simulink model "Model_Excel"  (R2020a)
settings: Solver=VariableStepAuto  StartTime=0.0  StopTime=inf  RelTol=1e-3
model workspace (MAT data in the model file):
  WinSize = 16
  fc_bandpass = [0.05 0.25]
undefined symbols (not defined in the file or in its folder): A1, A104210, D1, P104210, W1, W104210
libraries: gtecHighspeedLib x1, dspsigops x1, dspfdesign x1, dspstat3 x1
(part 1 of 2)
settings Model: Creator=LAB-OREN3  LastModifiedBy=LAB-OREN3

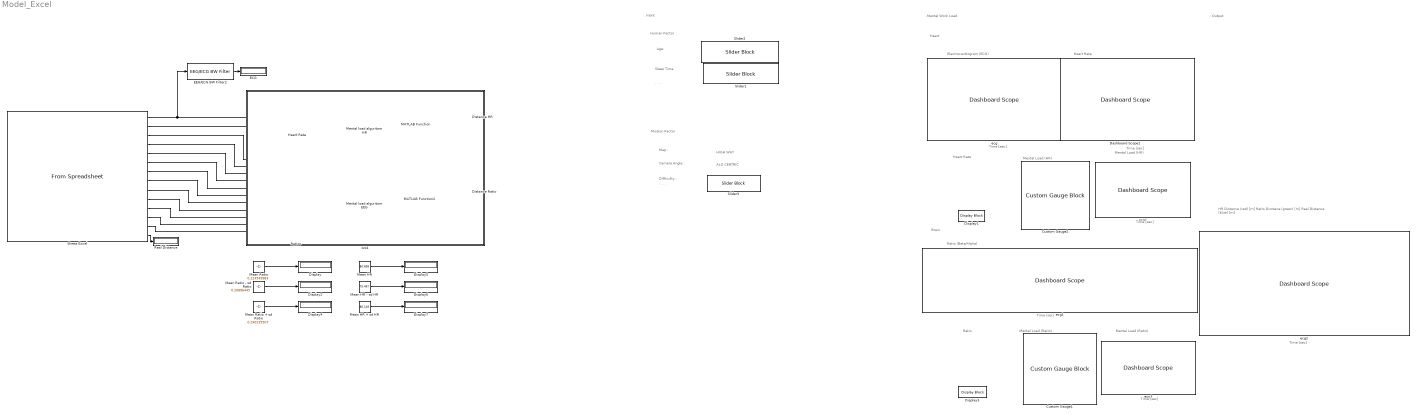
== system Model_Excel ==
  note: Time [sec]
  note: Heart Rate
  note: Mission Factor
  note: Ratio (Beta/Alpha)
  note: Electrocardiogram (ECG)
  note: Time (sec)
  note: Mental Load (Ratio)
  note: HIGH WAY
  note: Ratio
  note: ALO CENTRIC
  note: . Input
  note: Heart
  note: Time [sec]
  note: Sleep Time
  note: Human Factor
  note: Age:
  note: . Output
  note: Camera Angle: :
  note: . Mental Work Load
  note: Heart Rate
  note: Time [sec]
  note: Time [sec]
  note: Difficulty :
  note: .
      | .
      | .
      | .
  note: Brain
  note: Map :
  note: Time [sec]
  note: HR Distance (red) [m]
      | Ratio Disntace (green) [m]
      | Real Distance (blue) [m]
  note: .
      | .
      | .
      | .
  note: Mental Load (HR)
  note: Mental Load (Ratio)
  note: Mental Load (HR)
  Custom Gauge1 : CustomGaugeBlock  LabelPosition=Hide  NeedleImage=data:image/svg+xml;base64,PD94bWwgdmVyc2lvbj0iMS4wIiBlbmNvZGluZz0idXRmLTgiPz4KPCEtLSBHZW5lcmF0b3I6IEFkb2JlIElsbHVzdHJhdG9yIDE5LjIuMSwgU1ZHIEV4cG9ydCBQbHVnLUluIC4gU1ZHIFZlcnNpb246IDYuMDAgQnVpbGQgMCkgIC0tPgo8c3ZnIHZlcnNpb249IjEuMSIgeG1sbnM9Imh0dHA6Ly93d3cudzMub3JnLzIwMDAvc3ZnIiB4bWxuczp4bGluaz0iaHR0cDovL3d3dy53My5vcmcvMTk5OS94bGluayIgeD0iMHB4IiB5PSIwcHgiCgkgdmlld0JveD0iMCAwIDIwMCA1MCIgc3R5bGU9ImVuYWJsZS1iYWNrZ3JvdW5kOm5ldyAw ...(+9940 chars)  NeedleXPos=0.35442444142305646  NeedleYPos=0.4771166528829023  NeedleHeight=0.14101922133597494  NeedleWidth=0.2323187540223344  NeedleInitialRotation=-59.94322499147643  BackgroundImage=data:image/svg+xml;base64,PD94bWwgdmVyc2lvbj0iMS4wIiBlbmNvZGluZz0iVVRGLTgiIHN0YW5kYWxvbmU9Im5vIj8+CjwhLS0gR2VuZXJhdG9yOiBBZG9iZSBJbGx1c3RyYXRvciAxOS4yLjEsIFNWRyBFeHBvcnQgUGx1Zy1JbiAuIFNWRyBWZXJzaW9uOiA2LjAwIEJ1aWxkIDApICAtLT4KCjxzdmcKICAgeG1sbnM6ZGM9Imh0dHA6Ly9wdXJsLm9yZy9kYy9lbGVtZW50cy8xLjEvIgogICB4bWxuczpjYz0iaHR0cDovL2NyZWF0aXZlY29tbW9ucy5vcmcvbnMjIgogICB4bWxuczpyZGY9Imh0dHA6Ly93d3cudzMub3JnLzE5OTkvMDIvMjItcmRmLXN5bnRh ...(+9660 chars)  GaugeMax=1  GaugeArcDefined=true  GaugeArcRadius=0.16512766301399787  GaugeArcStrokeWidth=0.04828970295350007  GaugeArcRotation=240.5385250290321  GaugeArcRatio=0.8333333333333  GaugeArcTransparency=0  ValueArcTransparency=0  ValueArcColor=#1759b0  GaugeTickTransparency=0.55  GaugeTickColor=#faf5c8  ScaleColorsJSON="[{\"Min\":0,\"Max\":0.4,\"Color\":[0.39215686274509803,0.83137254901960778,0.074509803921568626]},{\"Min\":0.4,\"Max\":0.7,\"Color\":[0.92941176470588238,0.69411764705882351,0.12549019607843137]},{\"Min\":0.7,\"Max\":1,\"Color\":[0.996078431372549,0.2,0.0392156862745098]}]"  fixedAspectRatio=on  IsLinearGauge=false  GaugeTrackLeft=0.35  GaugeTrackTop=0.35  GaugeTrackHeight=0.1  GaugeTrackWidth=0.3  GaugeTrackRotation=0
  Custom Gauge2 : CustomGaugeBlock  LabelPosition=Hide  NeedleImage=data:image/svg+xml;base64,PD94bWwgdmVyc2lvbj0iMS4wIiBlbmNvZGluZz0idXRmLTgiPz4KPCEtLSBHZW5lcmF0b3I6IEFkb2JlIElsbHVzdHJhdG9yIDE5LjIuMSwgU1ZHIEV4cG9ydCBQbHVnLUluIC4gU1ZHIFZlcnNpb246IDYuMDAgQnVpbGQgMCkgIC0tPgo8c3ZnIHZlcnNpb249IjEuMSIgeG1sbnM9Imh0dHA6Ly93d3cudzMub3JnLzIwMDAvc3ZnIiB4bWxuczp4bGluaz0iaHR0cDovL3d3dy53My5vcmcvMTk5OS94bGluayIgeD0iMHB4IiB5PSIwcHgiCgkgdmlld0JveD0iMCAwIDIwMCA1MCIgc3R5bGU9ImVuYWJsZS1iYWNrZ3JvdW5kOm5ldyAw ...(+9940 chars)  NeedleXPos=0.3499172390096674  NeedleYPos=0.47640815567113937  NeedleHeight=0.14538535381695605  NeedleWidth=0.2395116348811877  NeedleInitialRotation=-59.94322499147643  BackgroundImage=data:image/svg+xml;base64,PD94bWwgdmVyc2lvbj0iMS4wIiBlbmNvZGluZz0iVVRGLTgiIHN0YW5kYWxvbmU9Im5vIj8+CjwhLS0gR2VuZXJhdG9yOiBBZG9iZSBJbGx1c3RyYXRvciAxOS4yLjEsIFNWRyBFeHBvcnQgUGx1Zy1JbiAuIFNWRyBWZXJzaW9uOiA2LjAwIEJ1aWxkIDApICAtLT4KCjxzdmcKICAgeG1sbnM6ZGM9Imh0dHA6Ly9wdXJsLm9yZy9kYy9lbGVtZW50cy8xLjEvIgogICB4bWxuczpjYz0iaHR0cDovL2NyZWF0aXZlY29tbW9ucy5vcmcvbnMjIgogICB4bWxuczpyZGY9Imh0dHA6Ly93d3cudzMub3JnLzE5OTkvMDIvMjItcmRmLXN5bnRh ...(+9660 chars)  GaugeMax=1  GaugeArcDefined=true  GaugeArcRadius=0.17024022317539741  GaugeArcStrokeWidth=0.04978481290067439  GaugeArcRotation=240.5385250290321  GaugeArcRatio=0.8333333333333  GaugeArcTransparency=0  ValueArcTransparency=0  ValueArcColor=#1759b0  GaugeTickColor=#faf5c8  ScaleColorsJSON="[{\"Min\":0,\"Max\":0.4,\"Color\":[0.39215686274509803,0.83137254901960778,0.074509803921568626]},{\"Min\":0.4,\"Max\":0.7,\"Color\":[0.92941176470588238,0.69411764705882351,0.12549019607843137]},{\"Min\":0.7,\"Max\":1,\"Color\":[0.996078431372549,0.2,0.0392156862745098]}]"  IsLinearGauge=false  GaugeTrackLeft=0.35  GaugeTrackTop=0.35  GaugeTrackHeight=0.1  GaugeTrackWidth=0.3  GaugeTrackRotation=0
  Dashboard Scope1 : DashboardScope  ShowInitialText=off  TimeSpan=50  Ymin=-1  Ymax=150  LegendPosition=Hide  ScaleAtStop=off
  Display{,2,4..7} (6 alike) : Display
  Display1 : DisplayBlock  LabelPosition=Hide  Format=bank  Transparency=1
  Display3 : DisplayBlock  LabelPosition=Hide  Format=short  Transparency=1
  Distance HR : Display
  Distance Ratio : Display
  ECG : Display
  EEG/ECG BW Filter2 : gtecHighspeedLib/EEG//ECG BW Filter  Order=6  LowerFreq=0.1  UpperFreq=30  SampFreq=512
      settings: SourceProductName=g.HIsys Library
  "Heart Rate " : Subsystem
  MATLAB Function : MATLAB Function  TreatAsAtomicUnit=on
  MATLAB Function2 : MATLAB Function  TreatAsAtomicUnit=on
  Mean HR : Constant  Value=80.808  VectorParams1D=off  SampleTime=0.5
  Mean HR + sd HR : Constant  Value=86.149  SampleTime=0.5
  Mean HR - sd HR : Constant  Value=75.467  SampleTime=0.5
  Mean Ratio : Constant  Value=0.224549983  VectorParams1D=off  SampleTime=0.5
  Mean Ratio + sd Ratio : Constant  Value=0.240135507  SampleTime=0.5
  Mean Ratio - sd Ratio : Constant  Value=0.20896445  SampleTime=0.5
  Mental load alguritom EEG : MATLAB Function  TreatAsAtomicUnit=on
  Mental load alguritom HR : MATLAB Function  TreatAsAtomicUnit=on
  Ratioo : Subsystem
  Real Distance : Display
  Slider1 : SliderBlock  LabelPosition=Hide  ScaleMax=10
  Slider2 : SliderBlock  LabelPosition=Hide  ScaleMin=10  ScaleMax=70  TickInterval=10
  Slider3 : SliderBlock  LabelPosition=Hide  ScaleMin=1  ScaleMax=3  TickInterval=1
  Stress Excel : FromSpreadsheet  FileName=C:\Users\LAB-OREN3\Desktop\CognataData\Participants_DATA\Ilan_Test\Physiological\Stress ilan at (13;34;7)\g.techAmp Data of Stress ilan at (13;34;7).xlsx  SheetName=גיליון1  Range=A1:A104210,D1:P104210,W1:W104210  SampleTime=0.001953125
  ecg : DashboardScope  Tag=ECG  ShowInitialText=off  TimeSpan=5  Ymin=-2500  Ymax=2500  LegendPosition=Hide  ScaleAtStop=off
  ecg1 : DashboardScope  Tag=ECG  ShowInitialText=off  TimeSpan=100  Ymin=0.15  Ymax=0.27  LegendPosition=Hide  ScaleAtStop=off
  ecg2 : DashboardScope  Tag=ECG  ShowInitialText=off  TimeSpan=50  Ymin=-1  Ymax=21  LegendPosition=Hide  ScaleAtStop=off
  ecg3 : DashboardScope  Tag=ECG  ShowInitialText=off  TimeSpan=50  Ymin=-0.1  Ymax=1.1  LegendPosition=Hide  ScaleAtStop=off
  ecg4 : DashboardScope  Tag=ECG  ShowInitialText=off  TimeSpan=50  Ymin=-0.1  Ymax=1.1  LegendPosition=Hide  ScaleAtStop=off
  zzz4 : Subsystem  TreatAsAtomicUnit=on
      settings: OpenFcn=% no-op
      mask Display: disp('')
  wires:
  MATLAB Function/1(y) -> Distance HR/1
  Ratioo/1(Mean_Ratio_multipul_ch) -> Mental load alguritom EEG/1(u)
  Mental load alguritom EEG/1(y) -> MATLAB Function2/1(u)
  MATLAB Function2/1(y) -> Distance Ratio/1
  Mental load alguritom HR/1(y) -> MATLAB Function/1(u)
  "Heart Rate "/1(Heat Rate 5 sec moving avrage) -> Mental load alguritom HR/1(u)
  Stress Excel/1 -> "Heart Rate "/1(In1), EEG/ECG BW Filter2/1
  EEG/ECG BW Filter2/1 -> ECG/1
  Stress Excel/14 -> Real Distance/1
  Stress Excel/2 -> Ratioo/1(In1)
  Stress Excel/3 -> Ratioo/2(In2)
  Stress Excel/4 -> Ratioo/3(In3)
  Stress Excel/5 -> Ratioo/4(In4)
  Stress Excel/6 -> Ratioo/5(In5)
  Stress Excel/7 -> Ratioo/6(In6)
  Stress Excel/8 -> Ratioo/7(In7)
  Stress Excel/9 -> Ratioo/8(In8)
  Stress Excel/10 -> Ratioo/9(In9)
  Stress Excel/11 -> Ratioo/10(In10)
  Stress Excel/12 -> Ratioo/11(In11)
  Stress Excel/13 -> Ratioo/12(In12)
  Mean Ratio/1 -> Display/1
  Mean Ratio - sd Ratio/1 -> Display2/1
  Mean Ratio + sd Ratio/1 -> Display4/1
  Mean HR + sd HR/1 -> Display7/1
  Mean HR/1 -> Display5/1
  Mean HR - sd HR/1 -> Display6/1

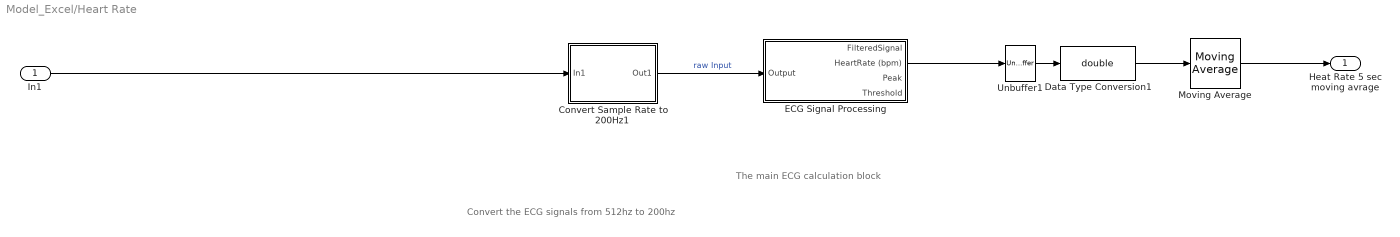
== system Model_Excel/Heart Rate  ==
  note: The main ECG calculation block
  note: Convert the ECG signals from 512hz to 200hz
  In1 : Inport
  Convert Sample Rate to 200Hz1 : Subsystem
  Data Type Conversion1 : DataTypeConversion  OutDataTypeStr=double
  ECG Signal Processing : Subsystem
  Moving Average : dspstat3/Moving Average  Method=Sliding window  ForgettingFactorPort=off  SpecifyWindowLength=on  WindowLength=1000  ForgettingFactor=0.9  SimulateUsing=Code generation
  Unbuffer1 : Unbuffer
  Heat Rate 5 sec moving avrage : Outport
  wires:
  In1/1 -> Convert Sample Rate to 200Hz1/1(In1)
  Unbuffer1/1 -> Data Type Conversion1/1
  Convert Sample Rate to 200Hz1/1(Out1) -> ECG Signal Processing/1(Output)  "raw Input"
  ECG Signal Processing/2(HeartRate (bpm)) -> Unbuffer1/1
  Data Type Conversion1/1 -> Moving Average/1
  Moving Average/1 -> Heat Rate 5 sec moving avrage/1

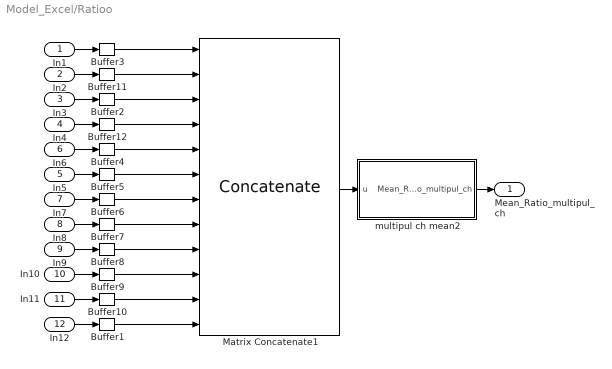
== system Model_Excel/Ratioo ==
  In1 : Inport
  In2 : Inport  Port=2
  In3 : Inport  Port=3
  In4 : Inport  Port=4
  In5 : Inport  Port=5
  In6 : Inport  Port=6
  In7 : Inport  Port=7
  In8 : Inport  Port=8
  In9 : Inport  Port=9
  In10 : Inport  Port=10
  In11 : Inport  Port=11
  In12 : Inport  Port=12
  Buffer{1..12} (12 alike) : Buffer  N=2560  V=2000  OutputFrames=off
  Matrix Concatenate1 : Concatenate  NumInputs=12  Mode=Multidimensional array  ConcatenateDimension=2
  multipul ch mean2 : MATLAB Function  TreatAsAtomicUnit=on
  Mean_Ratio_multipul_ch : Outport
  wires:
  Matrix Concatenate1/1 -> multipul ch mean2/1(u)
  Buffer8/1 -> Matrix Concatenate1/9
  Buffer10/1 -> Matrix Concatenate1/11
  Buffer6/1 -> Matrix Concatenate1/7
  Buffer2/1 -> Matrix Concatenate1/3
  Buffer5/1 -> Matrix Concatenate1/6
  Buffer4/1 -> Matrix Concatenate1/5
  Buffer9/1 -> Matrix Concatenate1/10
  In8/1 -> Buffer7/1
  In7/1 -> Buffer6/1
  Buffer7/1 -> Matrix Concatenate1/8
  In11/1 -> Buffer10/1
  In1/1 -> Buffer3/1
  In9/1 -> Buffer8/1
  In5/1 -> Buffer5/1
  multipul ch mean2/1(Mean_Ratio_multipul_ch) -> Mean_Ratio_multipul_ch/1
  In2/1 -> Buffer11/1
  In3/1 -> Buffer2/1
  In10/1 -> Buffer9/1
  In6/1 -> Buffer4/1
  In4/1 -> Buffer12/1
  In12/1 -> Buffer1/1
  Buffer1/1 -> Matrix Concatenate1/12
  Buffer3/1 -> Matrix Concatenate1/1
  Buffer11/1 -> Matrix Concatenate1/2
  Buffer12/1 -> Matrix Concatenate1/4
